simulink model "MicrostickII_ExternalMode"  (R2017b)
settings: Solver=FixedStepDiscrete  StartTime=0.0  StopTime=inf  FixedStep=0.01  RelTol=1e-3
undefined symbols (not defined in the file): A4, B0, B10, B11, B12, Max, MaxPer, ms, P20, P32, P42, P43, Pin, Resol, s, us
libraries: MCHP_Blockset x10
(part 2 of 2)

== system MicrostickII_ExternalMode/Sqrt ==
  In1 : Inport
  " Sqrt Q15" : Subsystem  TreatAsAtomicUnit=on
  "Sqrt Double - Reference " : Subsystem  TreatAsAtomicUnit=on
  Out1 : Outport  VectorParamsAs1DForOutWhenUnconnected=off
  Out2 : Outport  Port=2  VectorParamsAs1DForOutWhenUnconnected=off
  wires:
  In1/1 -> " Sqrt Q15"/1(In1), "Sqrt Double - Reference "/1(In1)
  " Sqrt Q15"/1(Out1) -> Out1/1
  "Sqrt Double - Reference "/1(Out2) -> Out2/1
  [Validation] -> "Sqrt Double - Reference "/Enable

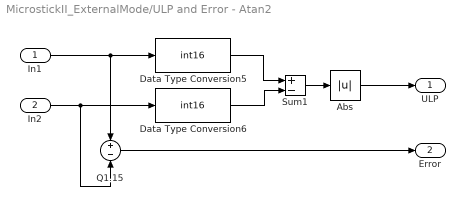
== system MicrostickII_ExternalMode/ULP and Error - Atan2 ==
  In1 : Inport
  In2 : Inport  Port=2
  Abs : Abs  SaturateOnIntegerOverflow=on
  Data Type Conversion5 : DataTypeConversion  OutDataTypeStr=int16  ConvertRealWorld=Stored Integer (SI)
  Data Type Conversion6 : DataTypeConversion  OutDataTypeStr=int16  ConvertRealWorld=Stored Integer (SI)
  Q1.15 : Sum  Inputs=+-  OutDataTypeStr=single
  Sum1 : Sum  Inputs=+-  SaturateOnIntegerOverflow=on  OutDataTypeStr=Inherit: Same as first input
  ULP : Outport  VectorParamsAs1DForOutWhenUnconnected=off
  Error : Outport  Port=2  VectorParamsAs1DForOutWhenUnconnected=off
  wires:
  Abs/1 -> ULP/1
  Q1.15/1 -> Error/1
  In1/1 -> Q1.15/1, Data Type Conversion5/1
  In2/1 -> Data Type Conversion6/1, Q1.15/2
  Sum1/1 -> Abs/1
  Data Type Conversion5/1 -> Sum1/1
  Data Type Conversion6/1 -> Sum1/2

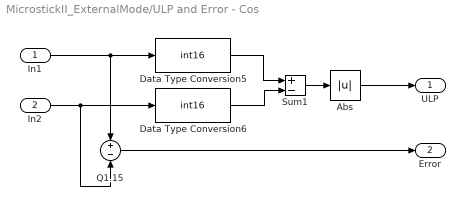
== system MicrostickII_ExternalMode/ULP and Error - Cos ==
  In1 : Inport
  In2 : Inport  Port=2
  Abs : Abs  SaturateOnIntegerOverflow=on
  Data Type Conversion5 : DataTypeConversion  OutDataTypeStr=int16  ConvertRealWorld=Stored Integer (SI)
  Data Type Conversion6 : DataTypeConversion  OutDataTypeStr=int16  ConvertRealWorld=Stored Integer (SI)
  Q1.15 : Sum  Inputs=+-  OutDataTypeStr=single
  Sum1 : Sum  Inputs=+-  SaturateOnIntegerOverflow=on  OutDataTypeStr=Inherit: Same as first input
  ULP : Outport  VectorParamsAs1DForOutWhenUnconnected=off
  Error : Outport  Port=2  VectorParamsAs1DForOutWhenUnconnected=off
  wires:
  Abs/1 -> ULP/1
  Q1.15/1 -> Error/1
  In1/1 -> Q1.15/1, Data Type Conversion5/1
  In2/1 -> Data Type Conversion6/1, Q1.15/2
  Sum1/1 -> Abs/1
  Data Type Conversion5/1 -> Sum1/1
  Data Type Conversion6/1 -> Sum1/2

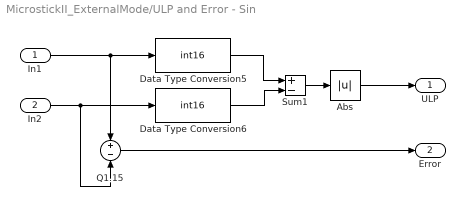
== system MicrostickII_ExternalMode/ULP and Error - Sin ==
  In1 : Inport
  In2 : Inport  Port=2
  Abs : Abs  SaturateOnIntegerOverflow=on
  Data Type Conversion5 : DataTypeConversion  OutDataTypeStr=int16  ConvertRealWorld=Stored Integer (SI)
  Data Type Conversion6 : DataTypeConversion  OutDataTypeStr=int16  ConvertRealWorld=Stored Integer (SI)
  Q1.15 : Sum  Inputs=+-  OutDataTypeStr=single
  Sum1 : Sum  Inputs=+-  SaturateOnIntegerOverflow=on  OutDataTypeStr=Inherit: Same as first input
  ULP : Outport  VectorParamsAs1DForOutWhenUnconnected=off
  Error : Outport  Port=2  VectorParamsAs1DForOutWhenUnconnected=off
  wires:
  Data Type Conversion6/1 -> Sum1/2
  Data Type Conversion5/1 -> Sum1/1
  Sum1/1 -> Abs/1
  In2/1 -> Q1.15/2, Data Type Conversion6/1
  In1/1 -> Data Type Conversion5/1, Q1.15/1
  Q1.15/1 -> Error/1
  Abs/1 -> ULP/1

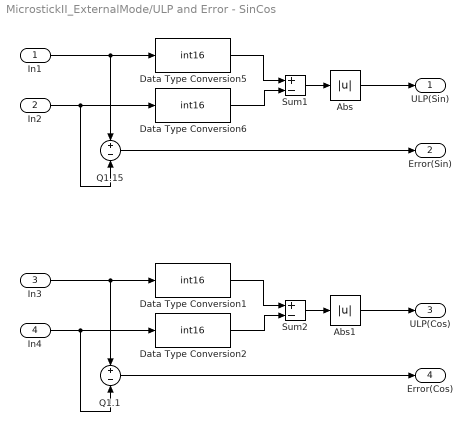
== system MicrostickII_ExternalMode/ULP and Error - SinCos ==
  In1 : Inport
  In2 : Inport  Port=2
  In3 : Inport  Port=3
  In4 : Inport  Port=4
  Abs : Abs  SaturateOnIntegerOverflow=on
  Abs1 : Abs  SaturateOnIntegerOverflow=on
  Data Type Conversion{1..2,5..6} (4 alike) : DataTypeConversion  OutDataTypeStr=int16  ConvertRealWorld=Stored Integer (SI)
  Q1.1 : Sum  Inputs=+-  OutDataTypeStr=single
  Q1.15 : Sum  Inputs=+-  OutDataTypeStr=single
  Sum1 : Sum  Inputs=+-  SaturateOnIntegerOverflow=on  OutDataTypeStr=Inherit: Same as first input
  Sum2 : Sum  Inputs=+-  SaturateOnIntegerOverflow=on  OutDataTypeStr=Inherit: Same as first input
  ULP(Sin) : Outport  VectorParamsAs1DForOutWhenUnconnected=off
  Error(Sin) : Outport  Port=2  VectorParamsAs1DForOutWhenUnconnected=off
  ULP(Cos) : Outport  Port=3  VectorParamsAs1DForOutWhenUnconnected=off
  Error(Cos) : Outport  Port=4  VectorParamsAs1DForOutWhenUnconnected=off
  wires:
  Data Type Conversion6/1 -> Sum1/2
  Data Type Conversion5/1 -> Sum1/1
  Sum1/1 -> Abs/1
  In2/1 -> Q1.15/2, Data Type Conversion6/1
  In1/1 -> Data Type Conversion5/1, Q1.15/1
  Q1.15/1 -> Error(Sin)/1
  Abs/1 -> ULP(Sin)/1
  Abs1/1 -> ULP(Cos)/1
  Q1.1/1 -> Error(Cos)/1
  In3/1 -> Q1.1/1, Data Type Conversion1/1
  In4/1 -> Data Type Conversion2/1, Q1.1/2
  Sum2/1 -> Abs1/1
  Data Type Conversion1/1 -> Sum2/1
  Data Type Conversion2/1 -> Sum2/2

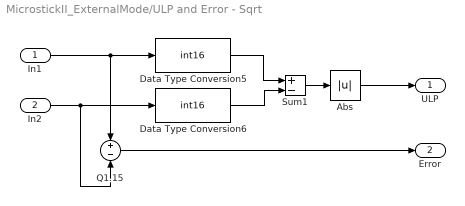
== system MicrostickII_ExternalMode/ULP and Error - Sqrt ==
  In1 : Inport
  In2 : Inport  Port=2
  Abs : Abs  SaturateOnIntegerOverflow=on
  Data Type Conversion5 : DataTypeConversion  OutDataTypeStr=int16  ConvertRealWorld=Stored Integer (SI)
  Data Type Conversion6 : DataTypeConversion  OutDataTypeStr=int16  ConvertRealWorld=Stored Integer (SI)
  Q1.15 : Sum  Inputs=+-  OutDataTypeStr=single
  Sum1 : Sum  Inputs=+-  SaturateOnIntegerOverflow=on  OutDataTypeStr=Inherit: Same as first input
  ULP : Outport  VectorParamsAs1DForOutWhenUnconnected=off
  Error : Outport  Port=2  VectorParamsAs1DForOutWhenUnconnected=off
  wires:
  Data Type Conversion6/1 -> Sum1/2
  Data Type Conversion5/1 -> Sum1/1
  Sum1/1 -> Abs/1
  In2/1 -> Q1.15/2, Data Type Conversion6/1
  In1/1 -> Data Type Conversion5/1, Q1.15/1
  Q1.15/1 -> Error/1
  Abs/1 -> ULP/1

== system MicrostickII_ExternalMode/Atan2/Atan2 Q15 ==
  In1 : Inport
  Atan2_Q1.15 : Subsystem  TreatAsAtomicUnit=on
  Demux : Demux  Outputs=2
  Out1 : Outport  VectorParamsAs1DForOutWhenUnconnected=off
  wires:
  Atan2_Q1.15/1(Out1) -> Out1/1
  Demux/1 -> Atan2_Q1.15/1(In1)
  Demux/2 -> Atan2_Q1.15/2(In2)
  In1/1 -> Demux/1

== system MicrostickII_ExternalMode/Atan2/Double Atan2 - Reference ==
  In1 : Inport
  Enable : EnablePort
  Demux : Demux  Outputs=2
  Simulink_Q1.15 : Subsystem  TreatAsAtomicUnit=on
  Simulink_Out_Q1.15 : Outport  VectorParamsAs1DForOutWhenUnconnected=off
  wires:
  Simulink_Q1.15/1(Out1) -> Simulink_Out_Q1.15/1
  In1/1 -> Demux/1
  Demux/1 -> Simulink_Q1.15/1(In1)
  Demux/2 -> Simulink_Q1.15/2(In2)

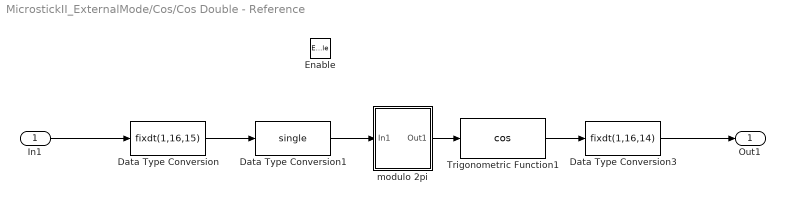
== system MicrostickII_ExternalMode/Cos/Cos Double - Reference ==
  In1 : Inport
  Enable : EnablePort
  Data Type Conversion : DataTypeConversion  OutDataTypeStr=fixdt(1,16,15)  ConvertRealWorld=Stored Integer (SI)
  Data Type Conversion1 : DataTypeConversion  OutDataTypeStr=single
  Data Type Conversion3 : DataTypeConversion  OutDataTypeStr=fixdt(1,16,14)  RndMeth=Convergent  SaturateOnIntegerOverflow=on
  Trigonometric Function1 : Trigonometry  Operator=cos  NumberOfIterations=15
  modulo 2pi : Subsystem
  Out1 : Outport  VectorParamsAs1DForOutWhenUnconnected=off
  wires:
  In1/1 -> Data Type Conversion/1
  Trigonometric Function1/1 -> Data Type Conversion3/1
  Data Type Conversion/1 -> Data Type Conversion1/1
  Data Type Conversion1/1 -> modulo 2pi/1(In1)
  modulo 2pi/1(Out1) -> Trigonometric Function1/1
  Data Type Conversion3/1 -> Out1/1

== system MicrostickII_ExternalMode/Cos/Cos Q15 ==
  In2 : Inport
  MCHP_Cos_Q1.15 : Subsystem  TreatAsAtomicUnit=on
  Cos_Out1 : Outport  OutDataTypeStr=fixdt(1,16,14)  VectorParamsAs1DForOutWhenUnconnected=off
  wires:
  In2/1 -> MCHP_Cos_Q1.15/1(In1)
  MCHP_Cos_Q1.15/1(Out1) -> Cos_Out1/1

== system MicrostickII_ExternalMode/Microstick2 - dsPIC33EP128MC202/1Hz Blinking2 ==
  Delay : Delay  DelayLength=1  InitialCondition=0  SampleTime=.5
  Logical Operator : Logic  Operator=NOT  AllPortsSameDT=off  OutDataTypeStr=boolean
  Rate Transition2 : RateTransition  Deterministic=off  OutPortSampleTime=.05
  Out1 : Outport  VectorParamsAs1DForOutWhenUnconnected=off
  wires:
  Delay/1 -> Logical Operator/1
  Logical Operator/1 -> Delay/1, Rate Transition2/1
  Rate Transition2/1 -> Out1/1

== system MicrostickII_ExternalMode/Microstick2 - dsPIC33EP128MC202/Open board doc WWW ==

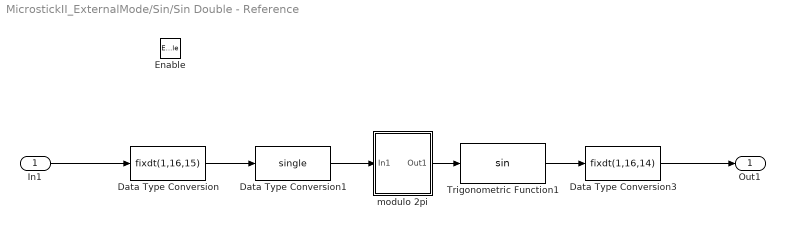
== system MicrostickII_ExternalMode/Sin/Sin Double - Reference ==
  In1 : Inport
  Enable : EnablePort
  Data Type Conversion : DataTypeConversion  OutDataTypeStr=fixdt(1,16,15)  ConvertRealWorld=Stored Integer (SI)
  Data Type Conversion1 : DataTypeConversion  OutDataTypeStr=single
  Data Type Conversion3 : DataTypeConversion  OutDataTypeStr=fixdt(1,16,14)  RndMeth=Convergent  SaturateOnIntegerOverflow=on
  Trigonometric Function1 : Trigonometry  NumberOfIterations=15
  modulo 2pi : Subsystem
  Out1 : Outport  VectorParamsAs1DForOutWhenUnconnected=off
  wires:
  Data Type Conversion3/1 -> Out1/1
  modulo 2pi/1(Out1) -> Trigonometric Function1/1
  Data Type Conversion1/1 -> modulo 2pi/1(In1)
  Data Type Conversion/1 -> Data Type Conversion1/1
  Trigonometric Function1/1 -> Data Type Conversion3/1
  In1/1 -> Data Type Conversion/1

== system MicrostickII_ExternalMode/Sin/Sin Q15 ==
  In2 : Inport
  MCHP_Sin_Q1.15 : Subsystem  TreatAsAtomicUnit=on
  Sin_Out1 : Outport  OutDataTypeStr=fixdt(1,16,14)  VectorParamsAs1DForOutWhenUnconnected=off
  wires:
  MCHP_Sin_Q1.15/1(Out1) -> Sin_Out1/1
  In2/1 -> MCHP_Sin_Q1.15/1(In1)

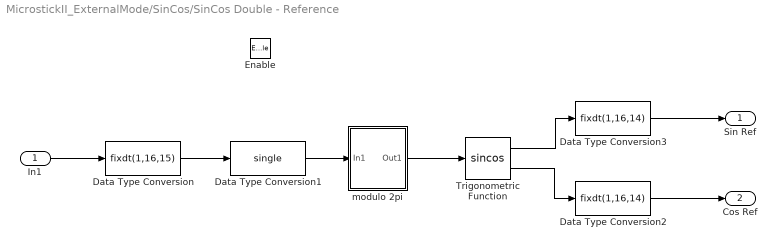
== system MicrostickII_ExternalMode/SinCos/SinCos Double - Reference ==
  In1 : Inport
  Enable : EnablePort
  Data Type Conversion : DataTypeConversion  OutDataTypeStr=fixdt(1,16,15)  ConvertRealWorld=Stored Integer (SI)
  Data Type Conversion1 : DataTypeConversion  OutDataTypeStr=single
  Data Type Conversion2 : DataTypeConversion  OutDataTypeStr=fixdt(1,16,14)  RndMeth=Convergent  SaturateOnIntegerOverflow=on
  Data Type Conversion3 : DataTypeConversion  OutDataTypeStr=fixdt(1,16,14)  RndMeth=Convergent  SaturateOnIntegerOverflow=on
  Trigonometric Function : Trigonometry  Operator=sincos
  modulo 2pi : Subsystem
  Sin Ref : Outport  VectorParamsAs1DForOutWhenUnconnected=off
  Cos Ref : Outport  Port=2  VectorParamsAs1DForOutWhenUnconnected=off
  wires:
  Data Type Conversion3/1 -> Sin Ref/1
  modulo 2pi/1(Out1) -> Trigonometric Function/1
  Data Type Conversion1/1 -> modulo 2pi/1(In1)
  Data Type Conversion/1 -> Data Type Conversion1/1
  Trigonometric Function/1 -> Data Type Conversion3/1
  In1/1 -> Data Type Conversion/1
  Data Type Conversion2/1 -> Cos Ref/1
  Trigonometric Function/2 -> Data Type Conversion2/1

== system MicrostickII_ExternalMode/SinCos/SinCos Q15 ==
  In2 : Inport
  MCHP_SinCos_Q1.15 : Subsystem  TreatAsAtomicUnit=on
  Sin_Out : Outport  OutDataTypeStr=fixdt(1,16,14)  VectorParamsAs1DForOutWhenUnconnected=off
  Cos_Out : Outport  Port=2  OutDataTypeStr=fixdt(1,16,14)  VectorParamsAs1DForOutWhenUnconnected=off
  wires:
  MCHP_SinCos_Q1.15/1(Out1) -> Sin_Out/1
  In2/1 -> MCHP_SinCos_Q1.15/1(In1)
  MCHP_SinCos_Q1.15/2(Out2) -> Cos_Out/1

== system MicrostickII_ExternalMode/Sqrt/ Sqrt Q15 ==
  In1 : Inport
  Sqrt : Sqrt  OutDataTypeStr=fixdt(1,16,15)
  Out1 : Outport  VectorParamsAs1DForOutWhenUnconnected=off
  wires:
  Sqrt/1 -> Out1/1
  In1/1 -> Sqrt/1

== system MicrostickII_ExternalMode/Sqrt/Sqrt Double - Reference  ==
  In1 : Inport
  Enable : EnablePort
  Data Type Conversion8 : DataTypeConversion  OutDataTypeStr=single
  Sqrt1 : Sqrt  OutDataTypeStr=fixdt(1,16,15)  RndMeth=Convergent
  Out2 : Outport  VectorParamsAs1DForOutWhenUnconnected=off
  wires:
  Sqrt1/1 -> Out2/1
  Data Type Conversion8/1 -> Sqrt1/1
  In1/1 -> Data Type Conversion8/1

== system MicrostickII_ExternalMode/Atan2/Atan2 Q15/Atan2_Q1.15 ==
  In1 : Inport
  In2 : Inport  Port=2
  Atan2 : Trigonometry  Operator=atan2  ApproximationMethod=CORDIC  NumberOfIterations=15  OutputSignalType=real
  Out1 : Outport  VectorParamsAs1DForOutWhenUnconnected=off
  wires:
  In1/1 -> Atan2/1
  In2/1 -> Atan2/2
  Atan2/1 -> Out1/1

== system MicrostickII_ExternalMode/Atan2/Double Atan2 - Reference/Simulink_Q1.15 ==
  In1 : Inport
  In2 : Inport  Port=2
  Data Type Conversion1 : DataTypeConversion  OutDataTypeStr=single
  Data Type Conversion3 : DataTypeConversion  OutDataTypeStr=single
  Data Type Conversion4 : DataTypeConversion  OutDataTypeStr=fixdt(1,16,13)  RndMeth=Convergent  SaturateOnIntegerOverflow=on
  Trigonometric Function1 : Trigonometry  Operator=atan2  NumberOfIterations=14  OutputSignalType=real
  Out1 : Outport  VectorParamsAs1DForOutWhenUnconnected=off
  wires:
  In2/1 -> Data Type Conversion3/1
  In1/1 -> Data Type Conversion1/1
  Data Type Conversion1/1 -> Trigonometric Function1/1
  Data Type Conversion3/1 -> Trigonometric Function1/2
  Trigonometric Function1/1 -> Data Type Conversion4/1
  Data Type Conversion4/1 -> Out1/1

== system MicrostickII_ExternalMode/Cos/Cos Double - Reference/modulo 2pi ==
  In1 : Inport
  Bias : Bias  Bias=pi
  Bias1 : Bias  Bias=-pi
  Constant2 : Constant  Value=2*pi  OutDataTypeStr=single  SampleTime=-1
  Math Function : Math  Operator=mod  SaturateOnIntegerOverflow=on
  Out1 : Outport  VectorParamsAs1DForOutWhenUnconnected=off
  wires:
  Bias1/1 -> Out1/1
  Bias/1 -> Math Function/1
  Constant2/1 -> Math Function/2
  Math Function/1 -> Bias1/1
  In1/1 -> Bias/1

== system MicrostickII_ExternalMode/Cos/Cos Q15/MCHP_Cos_Q1.15 ==
  In1 : Inport
  Cos : Trigonometry  Operator=cos  ApproximationMethod=CORDIC  NumberOfIterations=16
  Out1 : Outport  VectorParamsAs1DForOutWhenUnconnected=off
  wires:
  In1/1 -> Cos/1
  Cos/1 -> Out1/1

== system MicrostickII_ExternalMode/Sin/Sin Double - Reference/modulo 2pi ==
  In1 : Inport
  Bias : Bias  Bias=pi
  Bias1 : Bias  Bias=-pi
  Constant2 : Constant  Value=2*pi  OutDataTypeStr=single  SampleTime=-1
  Math Function : Math  Operator=mod  SaturateOnIntegerOverflow=on
  Out1 : Outport  VectorParamsAs1DForOutWhenUnconnected=off
  wires:
  In1/1 -> Bias/1
  Math Function/1 -> Bias1/1
  Constant2/1 -> Math Function/2
  Bias/1 -> Math Function/1
  Bias1/1 -> Out1/1

== system MicrostickII_ExternalMode/Sin/Sin Q15/MCHP_Sin_Q1.15 ==
  In1 : Inport
  Sin : Trigonometry  ApproximationMethod=CORDIC  NumberOfIterations=16
  Out1 : Outport  VectorParamsAs1DForOutWhenUnconnected=off
  wires:
  Sin/1 -> Out1/1
  In1/1 -> Sin/1

== system MicrostickII_ExternalMode/SinCos/SinCos Double - Reference/modulo 2pi ==
  In1 : Inport
  Bias : Bias  Bias=pi
  Bias1 : Bias  Bias=-pi
  Constant2 : Constant  Value=2*pi  OutDataTypeStr=single  SampleTime=-1
  Math Function : Math  Operator=mod  SaturateOnIntegerOverflow=on
  Out1 : Outport  VectorParamsAs1DForOutWhenUnconnected=off
  wires:
  In1/1 -> Bias/1
  Math Function/1 -> Bias1/1
  Constant2/1 -> Math Function/2
  Bias/1 -> Math Function/1
  Bias1/1 -> Out1/1

== system MicrostickII_ExternalMode/SinCos/SinCos Q15/MCHP_SinCos_Q1.15 ==
  In1 : Inport
  SinCos : Trigonometry  Operator=sincos  ApproximationMethod=CORDIC  NumberOfIterations=16
  Out1 : Outport  VectorParamsAs1DForOutWhenUnconnected=off
  Out2 : Outport  Port=2  VectorParamsAs1DForOutWhenUnconnected=off
  wires:
  SinCos/1 -> Out1/1
  In1/1 -> SinCos/1
  SinCos/2 -> Out2/1
